simulink library "RESET_LIB"  (R2021b)
settings: Solver=VariableStepAuto  StartTime=0.0  StopTime=10.0  RelTol=1e-3
settings Model: Creator=ACH  LastModifiedBy=ACH

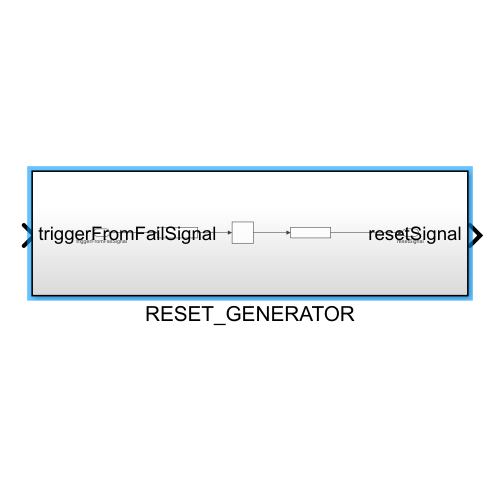
[thumbnail: Simulink's stored preview of the top-level diagram]
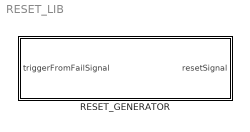
== system RESET_LIB ==
  RESET_GENERATOR : Subsystem

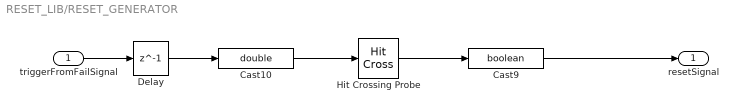
== system RESET_LIB/RESET_GENERATOR ==
  triggerFromFailSignal : Inport
  Cast10 : DataTypeConversion  OutDataTypeStr=double
  Cast9 : DataTypeConversion  OutDataTypeStr=boolean
  Delay : Delay  DelayLength=1
  Hit Crossing Probe : HitCross  HitCrossingOffset=0.5  HitCrossingDirection=falling
  resetSignal : Outport
  wires:
  Cast10/1 -> Hit Crossing Probe/1
  Hit Crossing Probe/1 -> Cast9/1
  triggerFromFailSignal/1 -> Delay/1
  Cast9/1 -> resetSignal/1
  Delay/1 -> Cast10/1
